simulink model "udp_send"  (R2014b)
settings: Solver=ode45  StartTime=0.0  StopTime=1.2  RelTol=1e-3
libraries: siglabs_lib x1, commrandsrc2 x1, dspnetwork x1
settings Model: NumberOfSteps=100  Creator=Ben  LastModifiedBy=Ben

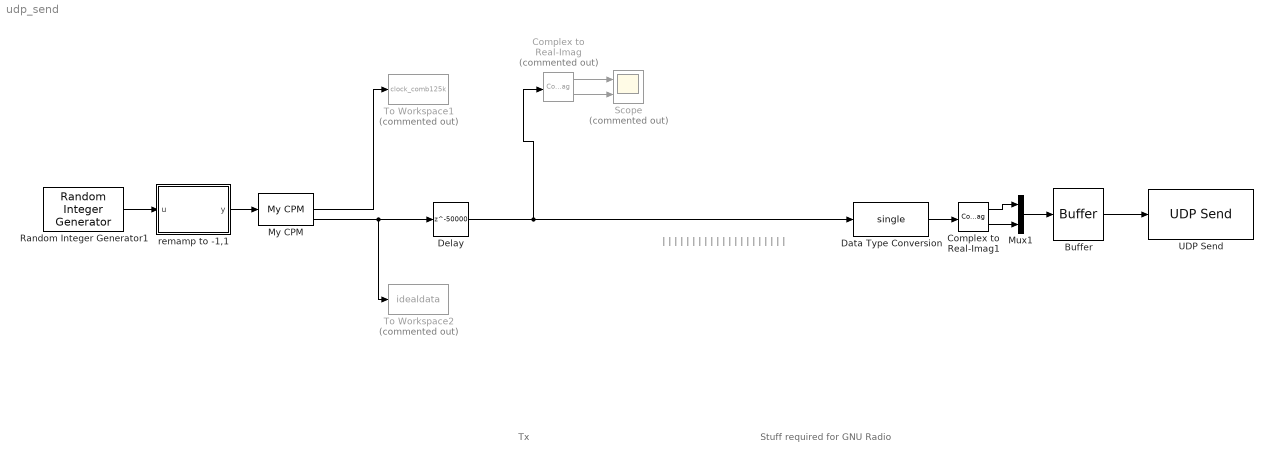
== system udp_send ==
  note: Stuff required for GNU Radio
  note: |
      | |
      | |
      | |
      | |
      | |
      | |
      | |
      | |
      | |
      | |
      | |
      | |
      | |
      | |
      | |
      | |
      | |
      | |
      | |
      | |
  note: Tx
  Buffer : Buffer  N=180  TreatMby1Signals=One channel
  Complex to Real-Imag : ComplexToRealImag  Commented=on
  Complex to Real-Imag1 : ComplexToRealImag
  Data Type Conversion : DataTypeConversion  OutDataTypeStr=single
  Delay : Delay  DelayLength=50000  InitialCondition=0
  Mux1 : Mux  Inputs=2
  My CPM : siglabs_lib/My CPM  SampsPerSym=50  RotationsPerSym=1  FilterBufferLength=3  ClockUpDownFrequency=100  PatternVectorDialog=[ones(1,7)*1 ones(1,7)*2 ones(1,6)*0]  PatternVectorRepeatDialog=2
  Random Integer Generator1 : commrandsrc2/Random Integer Generator  mul=2  seed=42  Ts=1/(2500)  frameBased=off  sampPerFrame=1024  orient=off  outDataType=double
  Scope : Scope  Commented=on  NumInputPorts=2
      settings: YMin=-5~-5  YMax=5~5
  To Workspace1 : ToWorkspace  Commented=on  VariableName=clock_comb125k  SampleTime=-1
      settings: Save2DSignal=2-D array (concatenate along first dimension)
  To Workspace2 : ToWorkspace  Commented=on  VariableName=idealdata  SampleTime=-1
      settings: Save2DSignal=2-D array (concatenate along first dimension)
  UDP Send : dspnetwork/UDP Send  remoteURL='192.168.1.24'  remotePort=1234  localURL='0.0.0.0'  localPortSource=Automatically determine  localPort=-1  sampletime=-1  separateLengthPort=0
  remamp to -1,1 : MATLAB Function  TreatAsAtomicUnit=on
  wires:
  Data Type Conversion/1 -> Complex to Real-Imag1/1
  Complex to Real-Imag1/1 -> Mux1/1
  Complex to Real-Imag1/2 -> Mux1/2
  Mux1/1 -> Buffer/1
  Buffer/1 -> UDP Send/1
  My CPM/3 -> To Workspace2/1, Delay/1
  Random Integer Generator1/1 -> remamp to -1,1/1(u)
  remamp to -1,1/1(y) -> My CPM/1
  Delay/1 -> Data Type Conversion/1, Complex to Real-Imag/1
  Complex to Real-Imag/1 -> Scope/1
  Complex to Real-Imag/2 -> Scope/2
  My CPM/2 -> To Workspace1/1

== matlab function udp_send/remamp to -1,1 ==
  data: u input; y output
function y = fcn(u)
%#codegen

y = (u*2)-1;
